simulink model "MSD"  (R2023a)
settings: Solver=VariableStepAuto  StartTime=0.0  StopTime=40  RelTol=1e-6
undefined symbols (not defined in the file): b, k, m
settings Model: Creator=Researcher  LastModifiedBy=Researcher

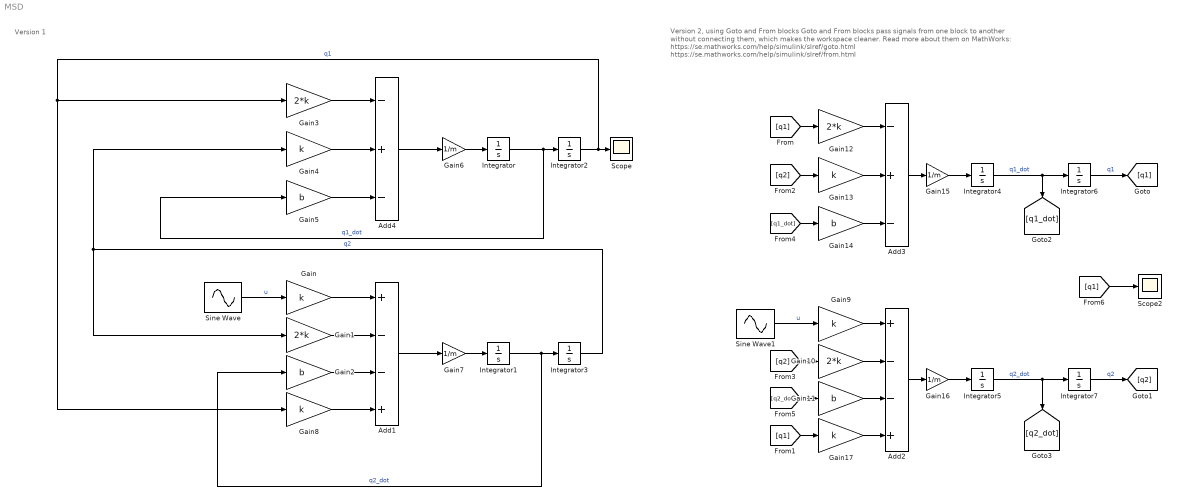
== system MSD ==
  note: Version 2, using Goto and From blocks
      | Goto and From blocks pass signals from one block to another without connecting them, which makes the workspace cleaner.
      | Read more about them on MathWorks:
      | https://se.mathworks.com/help/simulink/slref/goto.html
      | https://se.mathworks.com/help/simulink/slref/from.html
  note: Version 1
  Add1 : Sum  Inputs=+--+
  Add2 : Sum  Inputs=+--+
  Add3 : Sum  Inputs=-+-
  Add4 : Sum  Inputs=-+-
  Gain{,4,8..9,13,17} (6 alike) : Gain  Gain=k
  Gain{1,3,10,12} (4 alike) : Gain  Gain=2*k
  Gain{2,5,11,14} (4 alike) : Gain  Gain=b
  Gain{6..7,15..16} (4 alike) : Gain  Gain=1/m
  Integrator{,1..7} (8 alike) : Integrator
  Scope : Scope
  Scope2 : Scope
  Sine Wave : Sin  Amplitude=0.01  SampleTime=0
  Sine Wave1 : Sin  Amplitude=0.01  SampleTime=0
  wires:
  Sine Wave/1 -> Gain/1  "u"
  Gain/1 -> Add1/1
  Gain1/1 -> Add1/2
  Gain2/1 -> Add1/3
  Gain4/1 -> Add4/2
  Gain3/1 -> Add4/1
  Gain5/1 -> Add4/3
  Integrator3/1 -> Gain1/1, Gain4/1  "q2"
  Integrator/1 -> Gain5/1, Integrator2/1  "q1_dot"
  Add4/1 -> Gain6/1
  Add1/1 -> Gain7/1
  Gain8/1 -> Add1/4
  Integrator2/1 -> Scope/1, Gain3/1, Gain8/1  "q1"
  Gain6/1 -> Integrator/1
  Gain7/1 -> Integrator1/1
  Integrator1/1 -> Gain2/1, Integrator3/1  "q2_dot"
  Gain17/1 -> Add2/4
  Integrator5/1 -> Integrator7/1, [q2_dot]  "q2_dot"
  Add3/1 -> Gain15/1
  Integrator6/1 -> [q1]  "q1"
  Gain15/1 -> Integrator4/1
  Sine Wave1/1 -> Gain9/1  "u"
  Integrator4/1 -> Integrator6/1, [q1_dot]  "q1_dot"
  Gain13/1 -> Add3/2
  Integrator7/1 -> [q2]  "q2"
  Gain14/1 -> Add3/3
  Gain11/1 -> Add2/3
  Gain12/1 -> Add3/1
  Gain16/1 -> Integrator5/1
  Gain10/1 -> Add2/2
  Add2/1 -> Gain16/1
  Gain9/1 -> Add2/1
  [q1] -> Gain12/1
  [q1] -> Gain17/1
  [q2] -> Gain13/1
  [q2] -> Gain10/1
  [q1_dot] -> Gain14/1
  [q2_dot] -> Gain11/1
  [q1] -> Scope2/1
